simulink model "pendulum_aranya"  (Simulink 8.5)
settings: Solver=ode45  StartTime=0.0  StopTime=10.0  RelTol=1e-3
libraries: simulink x2
settings Model: Creator=Aranya Dan  LastModifiedBy=Aranya Dan
settings DataIOCC: SignalLoggingSaveFormat=Dataset
settings OptimizationCC: ExpressionDepthLimit=128
settings DebuggingCC: UnderspecifiedInitializationDetection=Simplified  MergeDetectMultiDrivingBlocksExec=error  FcnCallInpInsideContextMsg=EnableAllAsError  StateNameClashWarn=none
settings GRTTargetCC: CombineOutputUpdateFcns=on  GRTInterface=off

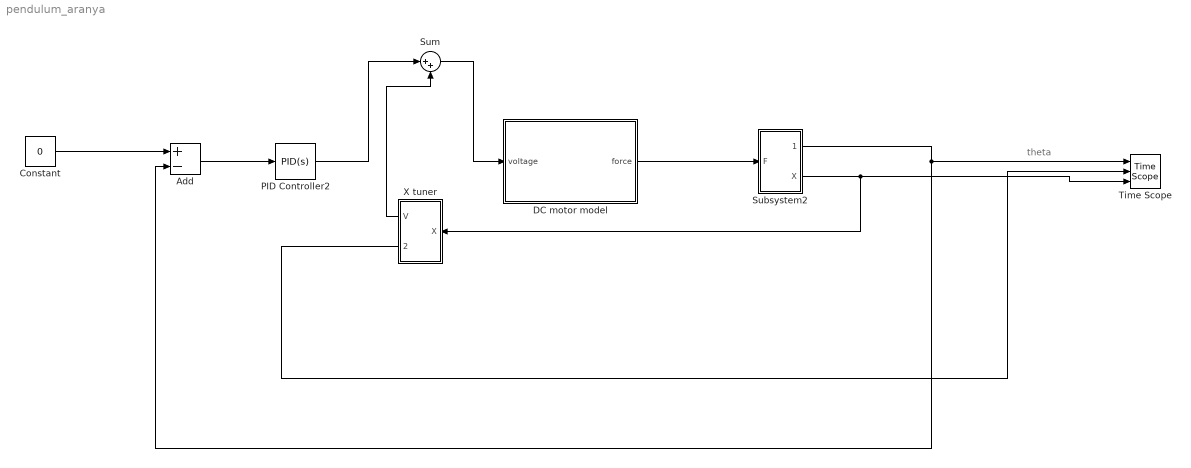
== system pendulum_aranya ==
  note: theta
  Add : Sum  Inputs=+-
  Constant : Constant  Value=0
  DC motor model : Subsystem
  PID Controller2 : simulink/Continuous/PID Controller  Controller=PID  TimeDomain=Continuous-time  SampleTime=-1  IntegratorMethod=Forward Euler  FilterMethod=Forward Euler  Form=Parallel  UseFilter=on  ControllerParametersSource=internal  P=185.474230733501  I=0.149570338875648  D=826.40709745591  N=0.0504202201249579  InitialConditionSource=internal  InitialConditionForIntegrator=0  InitialConditionForFilter=0  ExternalReset=none  LimitOutput=off  UpperSaturationLimit=inf  LowerSaturationLimit=-inf  LinearizeAsGain=off  AntiWindupMode=none  Kb=1  TrackingMode=off  Kt=1  PParamMin=[]  PParamMax=[]  IParamMin=[]  IParamMax=[]  DParamMin=[]  DParamMax=[]  NParamMin=[]  NParamMax=[]  KbParamMin=[]  KbParamMax=[]  KtParamMin=[]  KtParamMax=[]  POutMin=[]  POutMax=[]  IOutMin=[]  IOutMax=[]  DOutMin=[]  DOutMax=[]  NOutMin=[]  NOutMax=[]  KbOutMin=[]  KbOutMax=[]  KtOutMin=[]  KtOutMax=[]  IntegratorOutMin=[]  IntegratorOutMax=[]  FilterOutMin=[]  FilterOutMax=[]  SumOutMin=[]  SumOutMax=[]  SumI1OutMin=[]  SumI1OutMax=[]  SumI2OutMin=[]  SumI2OutMax=[]  SumI3OutMin=[]  SumI3OutMax=[]  SumDOutMin=[]  SumDOutMax=[]  SaturationOutMin=[]  SaturationOutMax=[]  IntegratorContinuousStateAttributes=''  IntegratorStateMustResolveToSignalObject=off  IntegratorRTWStateStorageClass=Auto  FilterContinuousStateAttributes=''  FilterStateMustResolveToSignalObject=off  FilterRTWStateStorageClass=Auto  DifferentiatorICPrevScaledInput=0  DifferentiatorOutMin=[]  DifferentiatorOutMax=[]
  Subsystem2 : Subsystem
  Sum : Sum  Inputs=|++
  Time Scope : TimeScope  DefaultConfigurationName=spbscopes.TimeScopeBlockCfg  NumInputPorts=3
  X tuner : Subsystem
  wires:
  Sum/1 -> DC motor model/1(voltage)
  Add/1 -> PID Controller2/1
  Constant/1 -> Add/1
  PID Controller2/1 -> Sum/1
  Subsystem2/1(theta) -> Add/2, Time Scope/1
  DC motor model/1(force) -> Subsystem2/1(F)
  X tuner/1(V) -> Sum/2
  X tuner/2(X des) -> Time Scope/2
  Subsystem2/2(X) -> X tuner/1(X), Time Scope/3

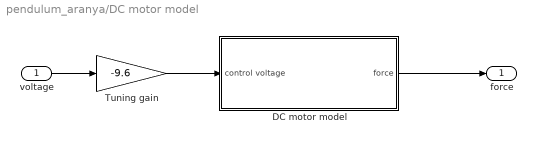
== system pendulum_aranya/DC motor model ==
  voltage : Inport
  DC motor model : Subsystem  mask{J=0.0000140, Kt=0.05, Kb=0.05, d=0.000001, R=2.5, L=0.0025}
      mask prompts: J "Moment of inertia"; Kt "Torque constant"; Kb "Electromotive force constant"; d "Linear approximation of viscous friction"; R "Electrical circuit resistance"; L "Electrical circuit inductance"
      mask Display: disp('DC motor')
  Tuning gain : Gain  Gain=-9.6
  force : Outport
  wires:
  Tuning gain/1 -> DC motor model/1(control voltage)
  voltage/1 -> Tuning gain/1
  DC motor model/1(force) -> force/1

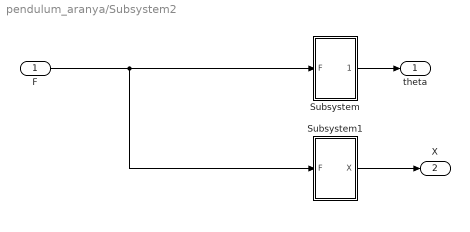
== system pendulum_aranya/Subsystem2 ==
  F : Inport
  Subsystem : Subsystem
  Subsystem1 : Subsystem
  theta : Outport
  X : Outport  Port=2
  wires:
  Subsystem/1(theta) -> theta/1
  F/1 -> Subsystem1/1(F), Subsystem/1(F)
  Subsystem1/1(X) -> X/1

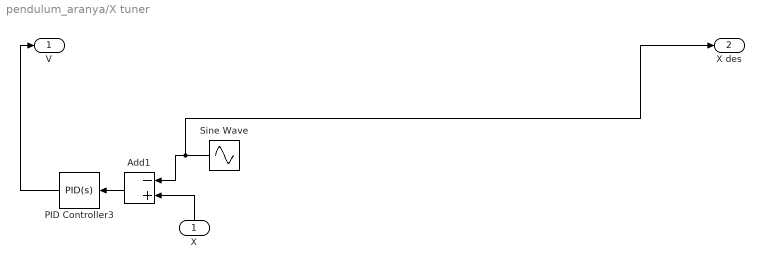
== system pendulum_aranya/X tuner ==
  X : Inport
  Add1 : Sum  Inputs=-+
  PID Controller3 : simulink/Continuous/PID Controller  Controller=PID  TimeDomain=Continuous-time  SampleTime=-1  IntegratorMethod=Forward Euler  FilterMethod=Forward Euler  Form=Parallel  UseFilter=on  ControllerParametersSource=internal  P=831.140160718589  I=29249.2650914478  D=5.88987419538334  N=29549.3786820731  InitialConditionSource=internal  InitialConditionForIntegrator=0  InitialConditionForFilter=0  ExternalReset=none  LimitOutput=off  UpperSaturationLimit=inf  LowerSaturationLimit=-inf  LinearizeAsGain=off  AntiWindupMode=none  Kb=1  TrackingMode=off  Kt=1  PParamMin=[]  PParamMax=[]  IParamMin=[]  IParamMax=[]  DParamMin=[]  DParamMax=[]  NParamMin=[]  NParamMax=[]  KbParamMin=[]  KbParamMax=[]  KtParamMin=[]  KtParamMax=[]  POutMin=[]  POutMax=[]  IOutMin=[]  IOutMax=[]  DOutMin=[]  DOutMax=[]  NOutMin=[]  NOutMax=[]  KbOutMin=[]  KbOutMax=[]  KtOutMin=[]  KtOutMax=[]  IntegratorOutMin=[]  IntegratorOutMax=[]  FilterOutMin=[]  FilterOutMax=[]  SumOutMin=[]  SumOutMax=[]  SumI1OutMin=[]  SumI1OutMax=[]  SumI2OutMin=[]  SumI2OutMax=[]  SumI3OutMin=[]  SumI3OutMax=[]  SumDOutMin=[]  SumDOutMax=[]  SaturationOutMin=[]  SaturationOutMax=[]  IntegratorContinuousStateAttributes=''  IntegratorStateMustResolveToSignalObject=off  IntegratorRTWStateStorageClass=Auto  FilterContinuousStateAttributes=''  FilterStateMustResolveToSignalObject=off  FilterRTWStateStorageClass=Auto  DifferentiatorICPrevScaledInput=0  DifferentiatorOutMin=[]  DifferentiatorOutMax=[]
  Sine Wave : Sin  SampleTime=0
  V : Outport
  X des : Outport  Port=2
  wires:
  Add1/1 -> PID Controller3/1
  PID Controller3/1 -> V/1
  Sine Wave/1 -> X des/1, Add1/1
  X/1 -> Add1/2

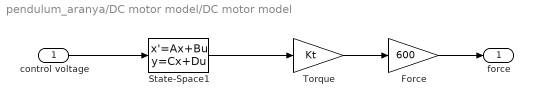
== system pendulum_aranya/DC motor model/DC motor model ==
  control voltage : Inport
  Force : Gain  Gain=600
  State-Space1 : StateSpace  A=[-d/J Kt/J;-Kb/L -R/L]  B=[0; 1/L]  C=[0 1]  D=0  X0=0
  Torque : Gain  Gain=Kt
  force : Outport
  wires:
  control voltage/1 -> State-Space1/1
  State-Space1/1 -> Torque/1
  Torque/1 -> Force/1
  Force/1 -> force/1

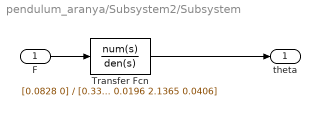
== system pendulum_aranya/Subsystem2/Subsystem ==
  F : Inport
  Transfer Fcn : TransferFcn  Numerator=[0.0828 0]  Denominator=[0.3319 0.0196 2.1365 0.0406]
  theta : Outport
  wires:
  F/1 -> Transfer Fcn/1
  Transfer Fcn/1 -> theta/1

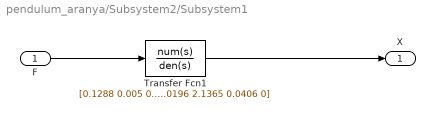
== system pendulum_aranya/Subsystem2/Subsystem1 ==
  F : Inport
  Transfer Fcn1 : TransferFcn  Numerator=[0.1288 0.005 0.8123]  Denominator=[0.3319 0.0196 2.1365 0.0406 0]
  X : Outport
  wires:
  F/1 -> Transfer Fcn1/1
  Transfer Fcn1/1 -> X/1
